simulink model "Non_coherent_demodulation"  (R2018b)
settings: Solver=VariableStepAuto  StartTime=0.0  StopTime=5e-2  RelTol=1e-3
libraries: dsparch4 x3, commchan3 x1
settings Model: Creator=sangh  LastModifiedBy=sangh

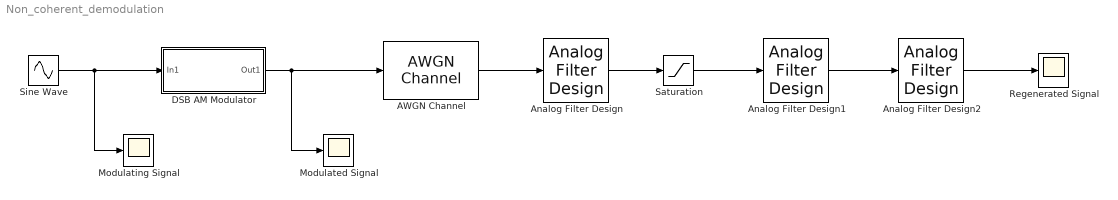
== system Non_coherent_demodulation ==
  AWGN Channel : commchan3/AWGN Channel  InputProcessing=Columns as channels (frame based)  seed=randseed  noiseMode=Variance from mask  EbNodB=10  EsNodB=10  SNRdB=10  bitsPerSym=1  Ps=1  Tsym=1  variance=0
  Analog Filter Design : dsparch4/Analog Filter Design  method=Butterworth  filttype=Bandpass  N=8  Wlo=2*pi*17e3  Whi=2*pi*23e3  Rp=2  Rs=40
  Analog Filter Design1 : dsparch4/Analog Filter Design  method=Butterworth  filttype=Lowpass  N=8  Wlo=2*pi*1000  Whi=80  Rp=2  Rs=40
  Analog Filter Design2 : dsparch4/Analog Filter Design  method=Butterworth  filttype=Highpass  N=8  Wlo=2*pi*200  Whi=80  Rp=2  Rs=40
  DSB AM Modulator : Subsystem
  Modulated Signal : Scope
  Modulating Signal : Scope
  Regenerated Signal : Scope
  Saturation : Saturate  UpperLimit=inf  LowerLimit=0
  Sine Wave : Sin  Frequency=2*pi*500  SampleTime=0.25e-6
  wires:
  AWGN Channel/1 -> Analog Filter Design/1
  Sine Wave/1 -> Modulating Signal/1, DSB AM Modulator/1(In1)
  DSB AM Modulator/1(Out1) -> AWGN Channel/1, Modulated Signal/1
  Analog Filter Design/1 -> Saturation/1
  Saturation/1 -> Analog Filter Design1/1
  Analog Filter Design1/1 -> Analog Filter Design2/1
  Analog Filter Design2/1 -> Regenerated Signal/1

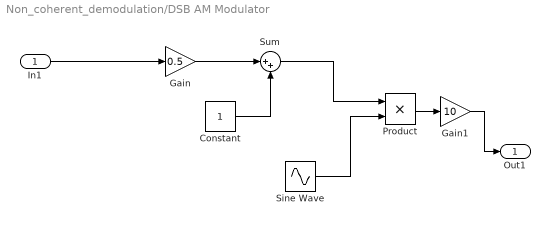
== system Non_coherent_demodulation/DSB AM Modulator ==
  In1 : Inport
  Constant : Constant
  Gain : Gain  Gain=0.5
  Gain1 : Gain  Gain=10
  Product : Product
  Sine Wave : Sin  Frequency=2*pi*20e3  SampleTime=0.25e-6
  Sum : Sum  Inputs=|++
  Out1 : Outport
  wires:
  In1/1 -> Gain/1
  Gain/1 -> Sum/1
  Constant/1 -> Sum/2
  Sine Wave/1 -> Product/2
  Sum/1 -> Product/1
  Product/1 -> Gain1/1
  Gain1/1 -> Out1/1
